simulink model "winch"  (R2020a)
settings: Solver=FixedStepAuto  StartTime=0.0  StopTime=1000  RelTol=1e-3
PreLoadFcn:
  | load("interfaces.mat");
  | load("winch_parameters.mat");
values from neighbouring files (symbols this model uses):
  K_d = 1000    [winch_parameters.mat]
  K_i = 1    [winch_parameters.mat]
  K_p = 200    [winch_parameters.mat]
libraries: simulink x1
settings Model: OrderedModelArguments=off  Creator=thomas.evang  LastModifiedBy=thomas.evang
settings RTWCC: Description=Generic Real-Time Target

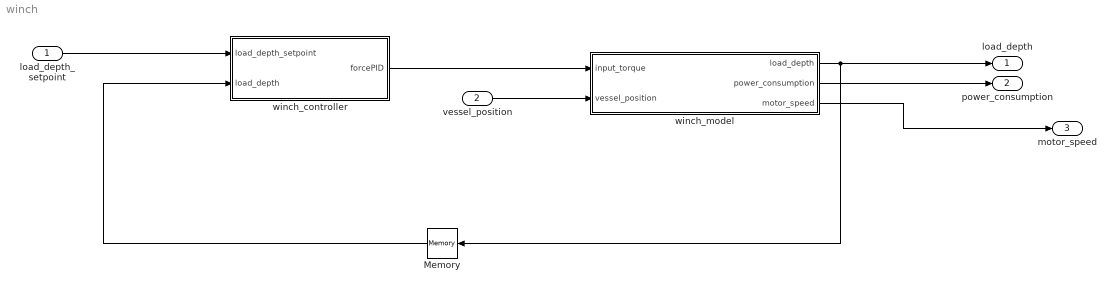
== system winch ==
  load_depth_setpoint : Inport
  vessel_position : Inport  Port=2  OutDataTypeStr=Bus: position_6dof
  Memory : Memory  InitialCondition=500
  winch_controller : Subsystem
  winch_model : Subsystem
  load_depth : Outport  VectorParamsAs1DForOutWhenUnconnected=off
  power_consumption : Outport  Port=2  VectorParamsAs1DForOutWhenUnconnected=off
  motor_speed : Outport  Port=3  VectorParamsAs1DForOutWhenUnconnected=off
  wires:
  vessel_position/1 -> winch_model/2(vessel_position)
  winch_model/1(load_depth) -> Memory/1, load_depth/1
  winch_model/2(power_consumption) -> power_consumption/1
  winch_model/3(motor_speed) -> motor_speed/1
  load_depth_setpoint/1 -> winch_controller/1(load_depth_setpoint)
  Memory/1 -> winch_controller/2(load_depth)
  winch_controller/1(forcePID) -> winch_model/1(input_torque)

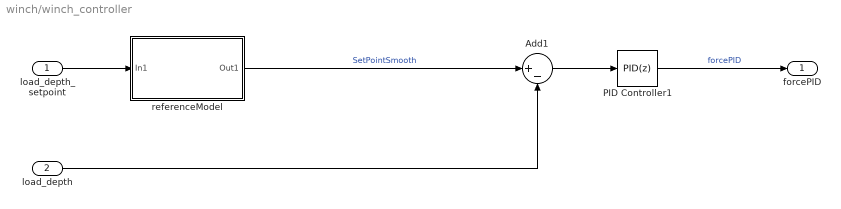
== system winch/winch_controller ==
  load_depth_setpoint : Inport
  load_depth : Inport  Port=2
  Add1 : Sum  Inputs=|+-
  PID Controller1 : simulink/Continuous/PID Controller  Controller=PID  Form=Parallel  TimeDomain=Discrete-time  UseExternalTs=off  SampleTime=1e-1  IntegratorMethod=Forward Euler  FilterMethod=Forward Euler  ControllerParametersSource=internal  P=K_p  I=K_i  D=K_d  UseFilter=off  N=100  TunerSelectOption=Transfer Function Based (PID Tuner App)  ZeroCross=off  InitialConditionSource=internal  InitialConditionForIntegrator=0  InitialConditionForFilter=0  DifferentiatorICPrevScaledInput=0  ExternalReset=none  TrackingMode=off  Kt=1  LimitOutput=off  UpperSaturationLimit=inf  LowerSaturationLimit=-inf  LinearizeAsGain=on  AntiWindupMode=none  Kb=1  POutMin=[]  POutMax=[]  IOutMin=[]  IOutMax=[]  DOutMin=[]  DOutMax=[]  NOutMin=[]  NOutMax=[]  SumOutMin=[]  SumOutMax=[]  SaturationOutMin=[]  SaturationOutMax=[]  PParamMin=[]  PParamMax=[]  IParamMin=[]  IParamMax=[]  DParamMin=[]  DParamMax=[]  NParamMin=[]  NParamMax=[]  KbParamMin=[]  KbParamMax=[]  KtParamMin=[]  KtParamMax=[]  KbOutMin=[]  KbOutMax=[]  KtOutMin=[]  KtOutMax=[]  IntegratorOutMin=[]  IntegratorOutMax=[]  FilterOutMin=[]  FilterOutMax=[]  SumI1OutMin=[]  SumI1OutMax=[]  SumI2OutMin=[]  SumI2OutMax=[]  SumI3OutMin=[]  SumI3OutMax=[]  SumI4OutMin=[]  SumI4OutMax=[]  SumDOutMin=[]  SumDOutMax=[]  DifferentiatorOutMin=[]  DifferentiatorOutMax=[]  FilterDiffOutCoefMin=[]  FilterDiffOutCoefMax=[]  ReciprocalOutMin=[]  ReciprocalOutMax=[]  SumDenOutMin=[]  SumDenOutMax=[]  SumNumOutMin=[]  SumNumOutMax=[]  DivideOutMin=[]  DivideOutMax=[]  UdiffTsProdOutMin=[]  UdiffTsProdOutMax=[]  NTsProdOutMin=[]  NTsProdOutMax=[]  UintegralTsProdOutMin=[]  UintegralTsProdOutMax=[]  UngainTsProdOutMin=[]  UngainTsProdOutMax=[]  IntegratorContinuousStateAttributes=''  IntegratorStateMustResolveToSignalObject=off  IntegratorRTWStateStorageClass=Auto  FilterContinuousStateAttributes=''  FilterStateMustResolveToSignalObject=off  FilterRTWStateStorageClass=Auto  ParallelPVariant=InternalParameters  IdealPVariant=Disabled  IVariant=InternalParameters  DVariant=InternalParameters  IntegratorVariant=Discrete  SatVariant=Disabled  AWVariant=Passthrough  PCopyVariant=Disabled  TRVariant=Disabled  FdbkBlocksVariant=Forward  IdealPFdbkVariant=Disabled  SatFdbkVariant=Disabled  DerivativeFilterVariant=Differentiator  NVariant=Passthrough  NCopyVariant=Disabled_SignalSpec  FilterICVariant=InternalICsDifferentiator  IntegratorICVariant=InternalICs  ExternalResetVariant=Disabled  TRSumVariant=Passthrough  SumFdbkVariant=Disabled  SumVariant=Sum_PID  TsampFilterVariant=InternalTs  TsampNgainVariant=Passthrough  TsampIntegralVariant=Passthrough
  referenceModel : Subsystem
  forcePID : Outport
  wires:
  referenceModel/1(Out1) -> Add1/1  "SetPointSmooth"
  Add1/1 -> PID Controller1/1
  PID Controller1/1 -> forcePID/1  "forcePID"
  load_depth_setpoint/1 -> referenceModel/1(In1)
  load_depth/1 -> Add1/2

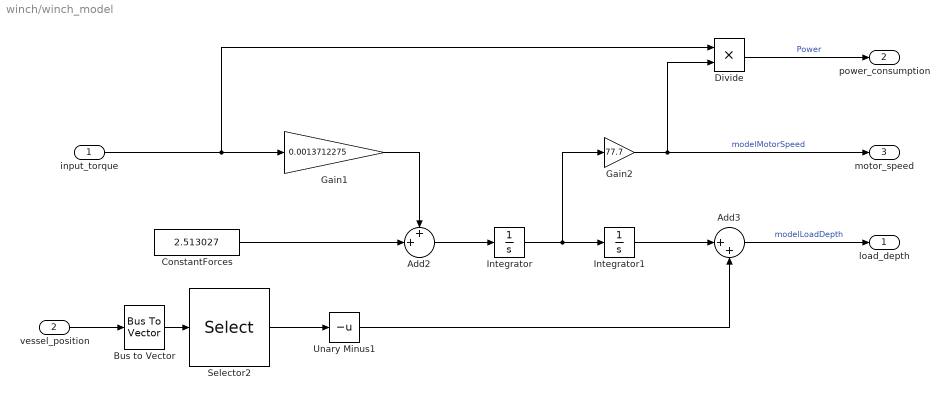
== system winch/winch_model ==
  input_torque : Inport  OutDataTypeStr=double
  vessel_position : Inport  Port=2  OutDataTypeStr=Bus: position_6dof
  Add2 : Sum  Inputs=++|
  Add3 : Sum  Inputs=|++
  Bus to Vector : BusToVector
  ConstantForces : Constant  Value=2.513027
  Divide : Product  Inputs=**
  Gain1 : Gain  Gain=0.0013712275
  Gain2 : Gain  Gain=77.7
  Integrator : Integrator
  Integrator1 : Integrator  InitialCondition=500
  Selector2 : Selector  InputPortWidth=6  IndexOptions=Index vector (dialog)  Indices=3  OutputSizes=1
  Unary Minus1 : UnaryMinus
  load_depth : Outport  VectorParamsAs1DForOutWhenUnconnected=off
  power_consumption : Outport  Port=2  VectorParamsAs1DForOutWhenUnconnected=off
  motor_speed : Outport  Port=3  VectorParamsAs1DForOutWhenUnconnected=off
  wires:
  Bus to Vector/1 -> Selector2/1
  Gain2/1 -> motor_speed/1, Divide/2  "modelMotorSpeed"
  ConstantForces/1 -> Add2/2
  Divide/1 -> power_consumption/1  "Power"
  input_torque/1 -> Divide/1, Gain1/1
  Gain1/1 -> Add2/1
  Integrator/1 -> Gain2/1, Integrator1/1
  Integrator1/1 -> Add3/1
  Add2/1 -> Integrator/1
  Selector2/1 -> Unary Minus1/1
  Unary Minus1/1 -> Add3/2
  vessel_position/1 -> Bus to Vector/1
  Add3/1 -> load_depth/1  "modelLoadDepth"

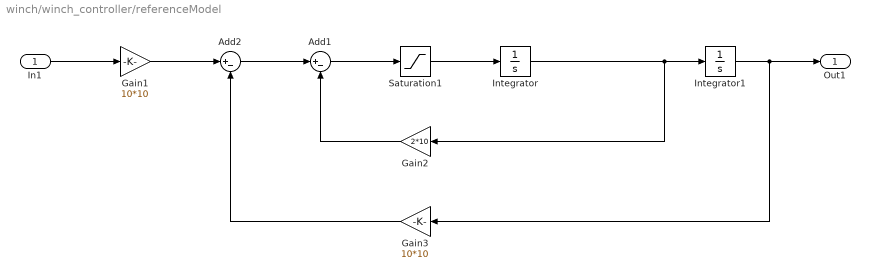
== system winch/winch_controller/referenceModel ==
  In1 : Inport
  Add1 : Sum  Inputs=|+-
  Add2 : Sum  Inputs=|+-
  Gain1 : Gain  Gain=10*10
  Gain2 : Gain  Gain=2*10
  Gain3 : Gain  Gain=10*10
  Integrator : Integrator  LimitOutput=on  UpperSaturationLimit=2  LowerSaturationLimit=-2  ZeroCross=off
  Integrator1 : Integrator  InitialCondition=500  ZeroCross=off
  Saturation1 : Saturate  UpperLimit=200  LowerLimit=-200  ZeroCross=off
  Out1 : Outport  VectorParamsAs1DForOutWhenUnconnected=off
  wires:
  In1/1 -> Gain1/1
  Gain1/1 -> Add2/1
  Add2/1 -> Add1/1
  Saturation1/1 -> Integrator/1
  Integrator1/1 -> Gain3/1, Out1/1
  Gain3/1 -> Add2/2
  Gain2/1 -> Add1/2
  Add1/1 -> Saturation1/1
  Integrator/1 -> Gain2/1, Integrator1/1
